simulink model "Quadrotor_SE3_Controller"  (R2023a)
settings: Solver=ode45  StartTime=0.0  StopTime=10  MaxStep=0.01  RelTol=1e-3
StopFcn:
  | close all
  | 
  | scale = 1;  % length of body axes arrows
  | 
  | % Body-frame axes arrows
  | H = 1;
  | Cviz = diag([1 1 -1]);
  | 
  | 
  | t = squeeze(out.tout);
  | R = squeeze(out.R_log.Data);
  | % Extract position
  | x = squeeze(out.x.Data);
  | y = squeeze(out.y.Data);
  | z = squeeze(out.z.Data);
  | 
  | xd = squeeze(out.xd.Data);
  | yd = squeeze(out.yd.Data);
  | zd = squeeze(out.zd.Data);
  | 
  | xv =  x;
  | yv =  y;
  | zv = -z;
  | 
  | xdv =  xd;
  | ydv =  yd;
  | zdv = -zd;
  | 
  | %
  | figure;
  | % plot3(x, y, z, 'b', 'LineWidth', 2);
  | grid on;
  | hold on;
  | view(3);
  | 
  | xlabel('X [m]');
  | ylabel('Y [m]');
  | zlabel('Z [m]');
  |  xlim([-1.25*H 1.25*H]);
  |  ylim([-1.25*H 1.25*H]);
  |  zlim([0 12.5*H]);
  | title('Quadrotor 3D Trajectory');
  | 
  | h = animatedline('LineWidth',2,'Color','b');
  | hd = animatedline('LineWidth',2,'Color','r');
  | 
  | 
  | p = plot3(x(1), y(1), z(1),'ko','MarkerFaceColor','g','MarkerSize',8);
  | pd = plot3(xd(1), yd(1), zd(1),'yo','MarkerFaceColor','k','MarkerSize',8);
  | 
  | qx = quiver3(x(1),y(1),z(1),0,0,0,'r','LineWidth',2);
  | qy = quiver3(x(1),y(1),z(1),0,0,0,'g','LineWidth',2);
  | qz = quiver3(x(1),y(1),z(1),0,0,0,'b','LineWidth',2);
  | 
  | % Initial time display
  | timeText = text(0, 0, 0, ...
  |     sprintf('t = %.2f s', t(1)), ...
  |     'FontSize',12, ...
  |     'FontWeight','bold', ...
  |     'BackgroundColor','w', ...
  |     'EdgeColor','k');
  | 
  | for k = 1:10:length(t)
  | 
  |     %Actual
  |     addpoints(h, xv(k), yv(k), zv(k))
  |     set(p, 'XData', xv(k), 'YData', yv(k), 'ZData', zv(k))
  | 
  |     % %Desired
  |     addpoints(hd, xdv(k), ydv(k), zdv(k))
  |     set(pd, 'XData', xdv(k), 'YData', ydv(k), 'ZData', zdv(k))
  | 
  |     Rk = reshape(R(:,k),3,3);
  |     Rviz = Cviz * Rk;
  | 
  |     % Body axes directions
  |     b1 = Rviz(:,1);
  |     b2 = Rviz(:,2);
  |     b3 = -Rviz(:,3);
  |     % Update arrows
  |     set(qx,'XData',xv(k),'YData',yv(k),'ZData',zv(k), ...
  |         'UData',scale*b1(1),'VData',scale*b1(2),'WData',scale*b1(3))
  | 
  |     set(qy,'XData',xv(k),'YData',yv(k),'ZData',zv(k), ...
  |         'UData',scale*b2(1),'VData',scale*b2(2),'WData',scale*b2(3))
  | 
  |     set(qz,'XData',xv(k),'YData',yv(k),'ZData',zv(k), ...
  |         'UData',scale*b3(1),'VData',scale*b3(2),'WData',scale*b3(3))
  | 
  | 
  |     set(timeText, ...
  |         'String', sprintf('t = %.2f s', t(k)), ...
  |         'Position', [1 -1 12])
  | 
  | 
  | 
  |     legend('Actual path','Desired Path','Actual Position','Desired Position');
  | 
  |     drawnow
  |     pause(0.1)
  | end
  | hold off;
  | 
  | 
  | 
  | 
  | 
  | % plot3(xd, yd, zd, 'LineWidth', 2);
  | % grid on;
  | hold off;
  | 
  | 
  | figure;
  | subplot(1,3,1)
  | plot(t,x);
  | hold on;
  | plot(t,xd);
  | legend('x','xd');
  | grid on
  | hold off;
  | ylabel('X [m]');
  | xlabel('Time [s]')
  | 
  | subplot(1,3,2)
  | plot(t,y);
  | hold on;
  | plot(t,yd);
  | legend('y','yd');
  | grid on
  | hold off;
  | ylabel('Y [m]');
  | xlabel('Time [s]')
  | 
  | subplot(1,3,3);
  | plot(t,z);
  | hold on;
  | plot(t,zd);
  | legend('z','zd');
  | grid on
  | hold off;
  | ylabel('Z [m]');
  | xlabel('Time [s]')
  | % axis ij;
settings Model: Creator=ttsm  LastModifiedBy=ttsm

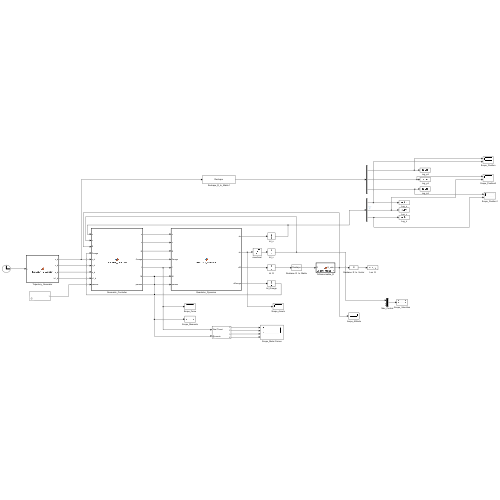
[thumbnail: Simulink's stored preview of the top-level diagram]
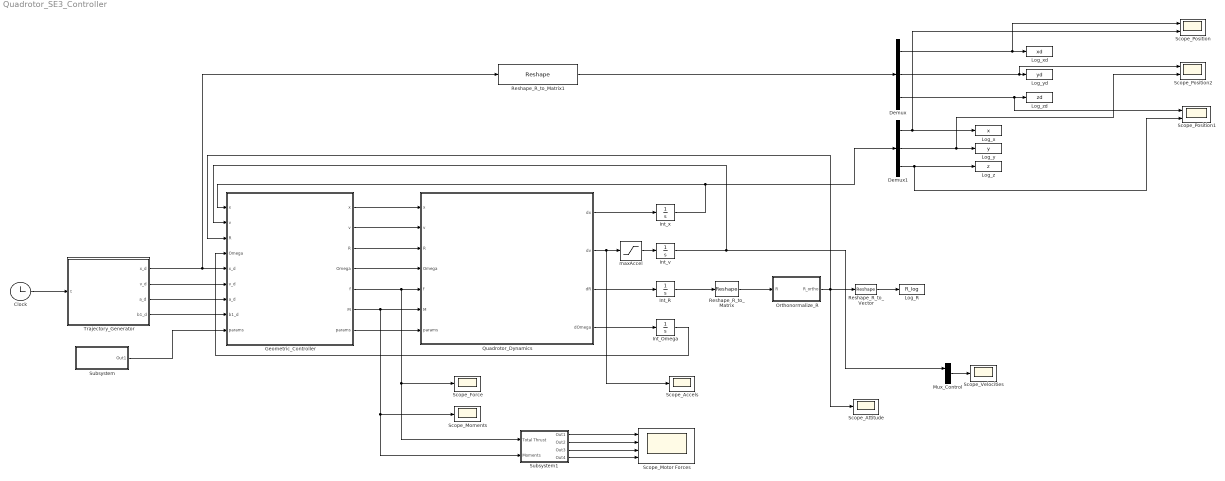
== system Quadrotor_SE3_Controller ==
  Clock : Clock
  Demux : Demux  Outputs=3
  Demux1 : Demux  Outputs=3
  Geometric_Controller : MATLAB Function  TreatAsAtomicUnit=on
  Int_Omega : Integrator  InitialCondition=[0;0;0]
  Int_R : Integrator  InitialCondition=reshape(diag([1;1;1]),9,1)
  Int_v : Integrator  InitialCondition=[0;0;0]
  Int_x : Integrator  InitialCondition=[0;0;0]
  Log_R : ToWorkspace  VariableName=R_log  SaveFormat=Timeseries  SampleTime=-1
  Log_x : ToWorkspace  VariableName=x  SaveFormat=Timeseries  SampleTime=-1
  Log_xd : ToWorkspace  VariableName=xd  SaveFormat=Timeseries  SampleTime=-1
  Log_y : ToWorkspace  VariableName=y  SaveFormat=Timeseries  SampleTime=-1
  Log_yd : ToWorkspace  VariableName=yd  SaveFormat=Timeseries  SampleTime=-1
  Log_z : ToWorkspace  VariableName=z  SaveFormat=Timeseries  SampleTime=-1
  Log_zd : ToWorkspace  VariableName=zd  SaveFormat=Timeseries  SampleTime=-1
  Mux_Control : Mux  Inputs=2
  Orthonormalize_R : MATLAB Function  TreatAsAtomicUnit=on
  Quadrotor_Dynamics : MATLAB Function  TreatAsAtomicUnit=on
  Reshape_R_to_Matrix : Reshape  OutputDimensionality=Customize  OutputDimensions=[3,3]
  Reshape_R_to_Matrix1 : Reshape  OutputDimensionality=Customize  OutputDimensions=[1,3]
  Reshape_R_to_Vector : Reshape  OutputDimensionality=Customize  OutputDimensions=[9,1]
  Scope_Accels : Scope
  Scope_Attitude : Scope
  Scope_Force : Scope
  Scope_Moments : Scope
  Scope_Motor Forces : Scope  NumInputPorts=4
  Scope_Position : Scope  NumInputPorts=2
  Scope_Position1 : Scope  NumInputPorts=2
  Scope_Position2 : Scope  NumInputPorts=2
  Scope_Velocities : Scope
  Subsystem : Subsystem  mask{m=4.34, g=9.81, k_x=2.3, k_v=2.1, k_R=16, k_Omega=1.7, Jxx=0.0820, Jyy=0.0854, Jzz=0.1377}
  Subsystem1 : Subsystem  mask{d=0.315, ct=0.008}
  Trajectory_Generator : MATLAB Function  TreatAsAtomicUnit=on
  maxAccel : Saturate  UpperLimit=maxSpeed  LowerLimit=-maxSpeed  mask{maxSpeed=5}
  wires:
  Clock/1 -> Trajectory_Generator/1(t)
  Quadrotor_Dynamics/4(dOmega) -> Int_Omega/1
  Int_R/1 -> Reshape_R_to_Matrix/1
  Reshape_R_to_Matrix/1 -> Orthonormalize_R/1(R)
  Orthonormalize_R/1(R_ortho) -> Scope_Attitude/1, Reshape_R_to_Vector/1, Geometric_Controller/3("R ")
  Int_x/1 -> Demux1/1, Geometric_Controller/1("x ")
  Trajectory_Generator/4(b1_d) -> Geometric_Controller/8(b1_d)
  Geometric_Controller/5(f) -> Subsystem1/1(Total Thrust), Scope_Force/1, Quadrotor_Dynamics/5(f)
  Geometric_Controller/6(M) -> Scope_Moments/1, Subsystem1/2(Moments), Quadrotor_Dynamics/6(M)
  Int_v/1 -> Geometric_Controller/2("v "), Mux_Control/1
  Int_Omega/1 -> Geometric_Controller/4("Omega ")
  Reshape_R_to_Vector/1 -> Log_R/1
  Quadrotor_Dynamics/3(dR) -> Int_R/1
  Trajectory_Generator/1(x_d) -> Reshape_R_to_Matrix1/1, Geometric_Controller/5(x_d)
  Reshape_R_to_Matrix1/1 -> Demux/1
  Mux_Control/1 -> Scope_Velocities/1
  Demux/1 -> Log_xd/1, Scope_Position/1
  Demux/2 -> Scope_Position2/1, Log_yd/1
  Demux/3 -> Scope_Position1/1, Log_zd/1
  Demux1/3 -> Scope_Position1/2, Log_z/1
  Demux1/2 -> Scope_Position2/2, Log_y/1
  Trajectory_Generator/2(v_d) -> Geometric_Controller/6(v_d)
  Trajectory_Generator/3(a_d) -> Geometric_Controller/7(a_d)
  Subsystem/1(Out1) -> Geometric_Controller/9("params ")
  Demux1/1 -> Scope_Position/2, Log_x/1
  Quadrotor_Dynamics/1(dx) -> Int_x/1
  Quadrotor_Dynamics/2(dv) -> Scope_Accels/1, maxAccel/1
  maxAccel/1 -> Int_v/1
  Geometric_Controller/1(x) -> Quadrotor_Dynamics/1(x)
  Geometric_Controller/2(v) -> Quadrotor_Dynamics/2(v)
  Geometric_Controller/3(R) -> Quadrotor_Dynamics/3(R)
  Geometric_Controller/4(Omega) -> Quadrotor_Dynamics/4(Omega)
  Geometric_Controller/7(params) -> Quadrotor_Dynamics/7(params)
  Subsystem1/1(Out1) -> Scope_Motor Forces/1
  Subsystem1/2(Out2) -> Scope_Motor Forces/2
  Subsystem1/3(Out3) -> Scope_Motor Forces/3
  Subsystem1/4(Out4) -> Scope_Motor Forces/4

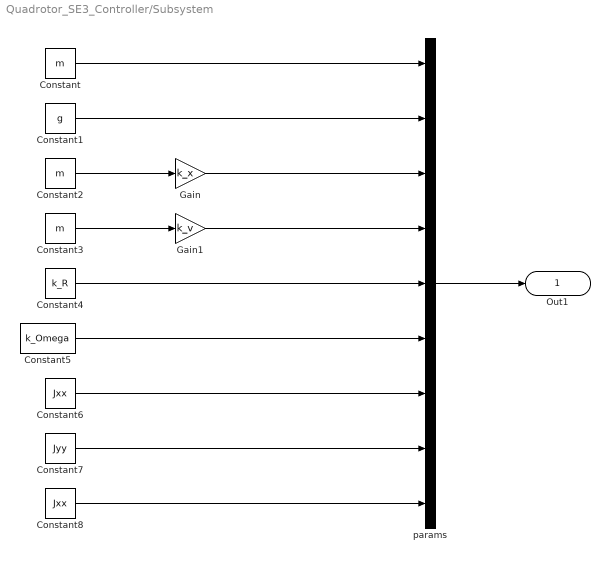
== system Quadrotor_SE3_Controller/Subsystem ==
  Constant : Constant  Value=m
  Constant1 : Constant  Value=g
  Constant2 : Constant  Value=m
  Constant3 : Constant  Value=m
  Constant4 : Constant  Value=k_R
  Constant5 : Constant  Value=k_Omega
  Constant6 : Constant  Value=Jxx
  Constant7 : Constant  Value=Jyy
  Constant8 : Constant  Value=Jxx
  Gain : Gain  Gain=k_x
  Gain1 : Gain  Gain=k_v
  params : Mux  Inputs=9
  Out1 : Outport
  wires:
  Constant6/1 -> params/7
  Constant7/1 -> params/8
  Constant8/1 -> params/9
  Constant5/1 -> params/6
  Constant4/1 -> params/5
  Constant3/1 -> Gain1/1
  Constant2/1 -> Gain/1
  Constant1/1 -> params/2
  Constant/1 -> params/1
  params/1 -> Out1/1
  Gain/1 -> params/3
  Gain1/1 -> params/4

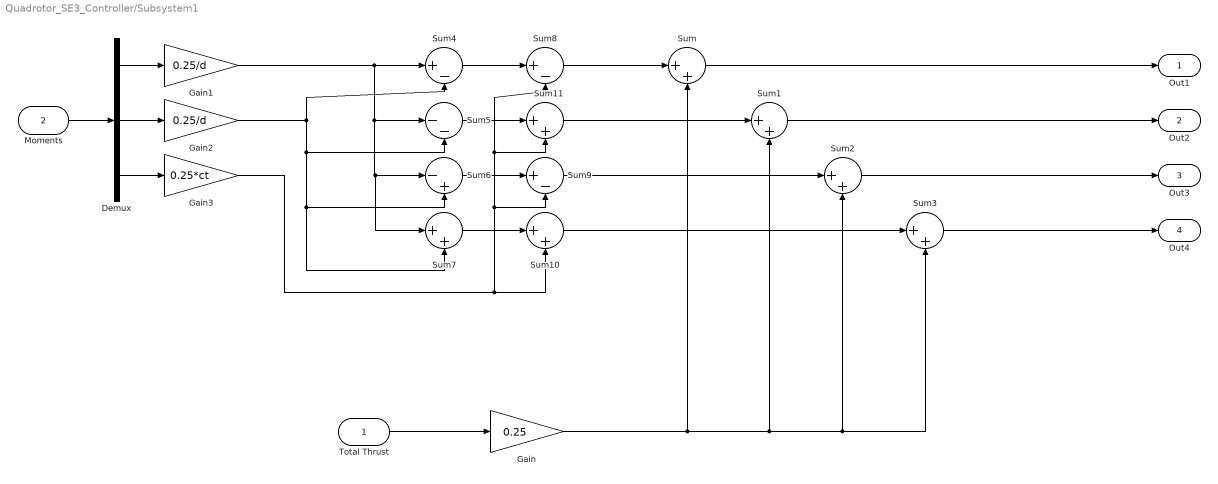
== system Quadrotor_SE3_Controller/Subsystem1 ==
  Total Thrust : Inport
  Moments : Inport  Port=2
  Demux : Demux  Outputs=3
  Gain : Gain  Gain=0.25
  Gain1 : Gain  Gain=0.25/d
  Gain2 : Gain  Gain=0.25/d
  Gain3 : Gain  Gain=0.25*ct
  Sum{,1..3,7,10..11} (7 alike) : Sum  Inputs=|++
  Sum4 : Sum  Inputs=|+-
  Sum5 : Sum  Inputs=|--
  Sum6 : Sum  Inputs=|-+
  Sum8 : Sum  Inputs=|+-
  Sum9 : Sum  Inputs=|+-
  Out1 : Outport
  Out2 : Outport  Port=2
  Out3 : Outport  Port=3
  Out4 : Outport  Port=4
  wires:
  Total Thrust/1 -> Gain/1
  Moments/1 -> Demux/1
  Demux/1 -> Gain1/1
  Demux/2 -> Gain2/1
  Demux/3 -> Gain3/1
  Gain/1 -> Sum/2, Sum1/2, Sum2/2, Sum3/2
  Sum/1 -> Out1/1
  Sum1/1 -> Out2/1
  Sum2/1 -> Out3/1
  Sum3/1 -> Out4/1
  Gain1/1 -> Sum5/1, Sum7/1, Sum6/1, Sum4/1
  Gain3/1 -> Sum8/2, Sum11/2, Sum9/2, Sum10/2
  Gain2/1 -> Sum5/2, Sum6/2, Sum7/2, Sum4/2
  Sum4/1 -> Sum8/1
  Sum5/1 -> Sum11/1
  Sum6/1 -> Sum9/1
  Sum7/1 -> Sum10/1
  Sum8/1 -> Sum/1
  Sum11/1 -> Sum1/1
  Sum9/1 -> Sum2/1
  Sum10/1 -> Sum3/1

== matlab function Quadrotor_SE3_Controller/Geometric_Controller ==
  data: x output; v output; R output; Omega output; x input; f output; v input; R input; Omega input; x_d input; v_d input; a_d input; b1_d input; M output; params input; params output
function [x,v,R,Omega,f, M,params] = Geometric_Controller(x, v, R, Omega, x_d, v_d, a_d, b1_d, params)
    % Extract parameters
    x = x;
    v = v;
    R = R;
    Omega = Omega;
    m = params(1); 
    g = params(2);
    k_x = params(3);
    k_v = params(4);
    k_R = params(5); 
    k_Omega = params(6);
    J = diag([params(7),params(8),params(9)]);
    e3 = [0; 0; 1];
    
    % Position tracking errors
    e_x = x - x_d; 
    e_v = v - v_d;
    
    % Desired thrust direction (Eq. 12)
    A = - k_x*e_x - k_v*e_v - m*g*e3 + m*a_d;
    A_norm = norm(A);
    if A_norm < 1e-6
        b3_d = -e3;
    else
        b3_d = -A / A_norm;
    end
    
    % Desired attitude
    b3_cross_b1 = cross(b3_d, b1_d);
    b3_cross_b1_norm = norm(b3_cross_b1);
    if b3_cross_b1_norm < 1e-6
        b2_d = [0; 1; 0];
        if abs(dot(b3_d, b2_d)) > 0.9, b2_d = [1; 0; 0]; end
        b2_d = cross(b3_d, b2_d); b2_d = b2_d / norm(b2_d);
    else
        b2_d = b3_cross_b1 / b3_cross_b1_norm;
    end
    b1_d_proj = cross(b2_d, b3_d);
    R_d = [b1_d_proj, b2_d, b3_d];
    
    % Total thrust (Eq. 15)
    f = -dot(A, R*e3);
    f = max(0,f);
    
    % Attitude errors (Eq. 10, 11)
    e_R_matrix = R_d' * R - R' * R_d;
    e_R = [e_R_matrix(3,2); e_R_matrix(1,3); e_R_matrix(2,1)] / 2;
    Omega_d = [0; 0; 0];
    Omega_d_dot = [0;0;0];
    e_Omega = Omega - R' * R_d * Omega_d;
    
    % Control moment (Eq. 16)
    Omega_hat = [0 -Omega(3) Omega(2); Omega(3) 0 -Omega(1); -Omega(2) Omega(1) 0];
    M = -k_R*e_R - k_Omega*e_Omega + cross(Omega, J*Omega) - J*(Omega_hat*R'*R_d*Omega_d - R'*R_d*Omega_d_dot);
    M = min(max(M, -5), 5);
end

== matlab function Quadrotor_SE3_Controller/Trajectory_Generator ==
  data: t input; x_d output; v_d output; a_d output; b1_d output
function [x_d,v_d,a_d,b1_d] = Trajectory_Generator(t)
    % Elliptical helix trajectory (Case I from paper)
    R = 1;
    w = pi/2;
    x_d = [R*cos(w*t); R*sin(w*t);-R*t];
    v_d = [-R*w*sin(w*t);R*w*cos(w*t);-R;];
    a_d = [-R*w^2*cos(w*t); -R*w^2*sin(w*t);0];
    % b1_d = [1;0;0];
    b1_d = [1; 0; 0];
    b1_d = b1_d / norm(b1_d);
end

% function [x_d, v_d, a_d, b1_d] = Trajectory_Generator(t)
%     % Simple L Trajectory with no yaw
%     R = 3;
%     if t >=1 && t<=5
%         x_d = [R;0;-R];
%         b1_d = [1; 0; 0];
% 
%     elseif t>5
%         x_d = [R;R;-R];
%         b1_d = [0; 1; 0];
% 
%     else 
%         x_d = [0;0;-R];
%         b1_d = [1; 0; 0];
% 
%     end
%     v_d = [0; 0; 0];
%     a_d = [0; 0; 0];
%     b1_d = b1_d / norm(b1_d);
% end

% function [x_d,v_d,a_d,b1_d] = Trajectory_Generator(t)
%     % Elliptical helix trajectory (Case I from paper)
%     R = 1;
%     w = pi/2;
%     x_d = [0;0;-5];
%     v_d = [0; 0; 0];
%     a_d = [0; 0; 0];
%     b1_d = [1;0;0];
%     % b1_d = [cos(w*t); sin(w*t); 0];
%     % b1_d = b1_d / norm(b1_d);
% end

== matlab function Quadrotor_SE3_Controller/Quadrotor_Dynamics ==
  data: x input; dx output; v input; R input; Omega input; f input; M input; params input; dv output; dR output; dOmega output
function [dx, dv, dR, dOmega] = Quadrotor_Dynamics(x, v, R, Omega, f, M, params)
    m = params(1); 
    g = params(2);
    J = diag([params(7),params(8),params(9)]);
    J_inv = inv(J);
    e3 = [0; 0; 1];
    % Translational dynamics (Eq. 2, 3)
    dx = v;
    dv = g*e3 - f/m*R*e3;


    
    % Rotational dynamics (Eq. 4, 5)
    Omega_hat = [0 -Omega(3) Omega(2); Omega(3) 0 -Omega(1); -Omega(2) Omega(1) 0];
    dRDot = R * Omega_hat;
    dR = reshape(dRDot,9,1);
    dOmega = J_inv*(-cross(Omega, J*Omega) + M);
end

== matlab function Quadrotor_SE3_Controller/Orthonormalize_R ==
  data: R input; R_ortho output
function R_ortho = Orthonormalize_R(R)
    % Gram-Schmidt orthonormalization
    b1 = R(:,1); b1 = b1 / norm(b1);
    b2 = R(:,2); b2 = b2 - dot(b2, b1)*b1; b2 = b2 / norm(b2);
    b3 = cross(b1, b2);
    R_ortho = [b1, b2, b3];
end
